simulink model "ICAR"  (R2018b)
settings: Solver=FixedStepAuto  StartTime=0.0  StopTime=10.0  RelTol=1e-3
(part 4 of 4)

== matlab function ICAR/ICAR/MATLAB Function1 ==
  data: y output
function y = fcn()

y = zeros(1,40);

== matlab function ICAR/ICAR/MATLAB Function ==
  data: y output
function y = fcn()

y = zeros(1,240);

== matlab function ICAR/ICAR/MATLAB Function3 ==
  data: y output
function y = fcn()

y = zeros(1,40);

== matlab function ICAR/ICAR/MATLAB Function4 ==
  data: y output
function y = fcn()

y = zeros(1,40);

== matlab function ICAR/ICAR/MATLAB Function5 ==
  data: y output
function y = fcn()

y = zeros(1,40);

== matlab function ICAR/ICAR/MATLAB Function6 ==
  data: y output
function y = fcn()

y = zeros(1,40);

== matlab function ICAR/ICAR/MATLAB Function7 ==
  data: y output
function y = fcn()

y = zeros(1,40);

== matlab function ICAR/ICAR/MATLAB Function8 ==
  data: y output
function y = fcn()

y = zeros(1,40);

== matlab function ICAR/ICAR/MATLAB Function9 ==
  data: y output
function y = fcn()

y = zeros(1,40);

== matlab function ICAR/ICAR/MATLAB Function10 ==
  data: y output
function y = fcn()

y = zeros(1,40);

== matlab function ICAR/ICAR/MATLAB Function11 ==
  data: y output
function y = fcn()

y = zeros(1,40);

== matlab function ICAR/ICAR/MATLAB Function12 ==
  data: y output
function y = fcn()

y = zeros(1,40);

== matlab function ICAR/ICAR/MATLAB Function13 ==
  data: y output
function y = fcn()

y = zeros(1,40);

== matlab function ICAR/ICAR/MATLAB Function14 ==
  data: y output
function y = fcn()

y = zeros(1,40);

== matlab function ICAR/ICAR/MATLAB Function15 ==
  data: y output
function y = fcn()

y = zeros(1,40);

== matlab function ICAR/ICAR/MATLAB Function16 ==
  data: y output
function y = fcn()

y = zeros(1,40);

== matlab function ICAR/ICAR/MATLAB Function17 ==
  data: y output
function y = fcn()

y = zeros(1,40);

== matlab function ICAR/ICAR/MATLAB Function18 ==
  data: y output
function y = fcn()

y = zeros(1,40);

== matlab function ICAR/ICAR/MATLAB Function19 ==
  data: y output
function y = fcn()

y = zeros(1,40);

== matlab function ICAR/ICAR/MATLAB Function20 ==
  data: y output
function y = fcn()

y = zeros(1,40);

== matlab function ICAR/ICAR/MATLAB Function21 ==
  data: y output
function y = fcn()

y = zeros(1,40);

== matlab function ICAR/ICAR/MATLAB Function22 ==
  data: y output
function y = fcn()

y = zeros(1,40);

== matlab function ICAR/ICAR/MATLAB Function23 ==
  data: y output
function y = fcn()

y = zeros(1,40);

== matlab function ICAR/ICAR/MATLAB Function24 ==
  data: y output
function y = fcn()

y = zeros(1,40);

== matlab function ICAR/ICAR/MATLAB Function25 ==
  data: y output
function y = fcn()

y = zeros(1,40);

== matlab function ICAR/ICAR/MATLAB Function26 ==
  data: y output
function y = fcn()

y = zeros(1,40);
